simulink model "TEST_IPM_2_0"  (R2019b)
settings: configuration reference "Configuration" (kept outside this file)
PreLoadFcn:
  | RTWConfigurationCB('preloadfcn', bdroot);
values from neighbouring files (symbols this model uses):
  MParamFbase = 200.0    [TEST_IPM_LIB.sldd]
  MParamIbase = 360.0    [TEST_IPM_LIB.sldd]
  MParamLd = 8.0E-5    [TEST_IPM_LIB.sldd]
  MParamLq = 0.00028    [TEST_IPM_LIB.sldd]
  MParamRs = 0.014    [TEST_IPM_LIB.sldd]
  PWM_TPBRD_HALF = 5000.0    [TEST_IPM_LIB.sldd]
  Ts_10kHz = 0.0001    [TEST_IPM_LIB.sldd]
  Ts_1kHz = 0.001    [TEST_IPM_LIB.sldd]
undefined symbols (not defined in the file or in its folder): DiscIntNeverNeededParam, Down, GPTRIP1SEL, GPTRIP2SEL, TZ1, TZ2, Up
libraries: c280xlib x24, c2837xDlib x18, dsparch4 x11, c2802xlib x10, powerlib_meascontrol x9, dspstat3 x2, c2000lib x1, c2806xlib x1, idelinklib_common x1
(part 6 of 6)

== matlab function TEST_IPM_2_0/INT/Data Buffer/MATLAB Function ==
  data: IdREF input; IdFBK input; UdComP input; IqREF input; IqFBK input; UqComP input; Theta input; ArrayId_REF data_store_memory; ArrayId_FBK data_store_memory; ArrayIq_REF data_store_memory; ArrayIq_FBK data_store_memory; ArrayUdComP data_store_memory; ArrayUqComP data_store_memory; ArrayTheta data_store_memory; BufferFlag data_store_memory
function Buffer_In(IdREF,IdFBK,UdComP,IqREF,IqFBK,UqComP,Theta)
global ArrayId_REF ArrayId_FBK ArrayUdComP 
global ArrayIq_REF ArrayIq_FBK ArrayUqComP
global ArrayTheta
global BufferFlag
persistent count
if isempty(count)
	count = uint16(1);
end

if(BufferFlag == 1)
    count = uint16(1);
else
    if(count <= uint16(500))
        ArrayId_REF(count) = single(IdREF);
        ArrayId_FBK(count) = single(IdFBK);
        ArrayUdComP(count) = single(UdComP);
        ArrayIq_REF(count) = single(IqREF);
        ArrayIq_FBK(count) = single(IqFBK);
        ArrayUqComP(count) = single(UqComP);
        ArrayTheta (count) = single(Theta);
        count = count + uint16(1);
    else
        count = uint16(1);
        BufferFlag = uint16(1);
    end
end
end

== stateflow chart TEST_IPM_2_0/INT/MAX5742/MAX5742 ==
  settings: updateMethod=DISCRETE  initializeOutput=1  enableNonTerminalStates=1
  state DAC_A
    entry:
    count_5742 = uint16(0);
    DAC_A_OUT();
  state Wait
    entry:
    count_5742 = count_5742 + uint16(1);
  state DAC_B
    entry:
    count_5742 = uint16(0);
    DAC_B_OUT();
  state empty
  state Wait1
    entry:
    count_5742 = count_5742 + uint16(1);
  state DAC_C
    entry:
    count_5742 = uint16(0);
    DAC_C_OUT();
  state Wait3
    entry:
    count_5742 = count_5742 + uint16(1);
  state DAC_D
    entry:
    FLAG_5742 = uint16(1);
    count_5742 = uint16(0);
    DAC_D_OUT();
  (default) -> DAC_A
  empty -> DAC_A : [FLAG_5742 == 0]
  DAC_A -> (junction 5)
  (junction 5) -> Wait [order 2]
  Wait -> (junction 5)
  (junction 5) -> DAC_B [order 1] : [count_5742 > 20]
  DAC_B -> (junction 15)
  DAC_D -> empty
  (junction 15) -> Wait1 [order 2]
  Wait1 -> (junction 15)
  (junction 15) -> DAC_C [order 1] : [count_5742 > 20]
  DAC_C -> (junction 34)
  (junction 34) -> Wait3 [order 2]
  Wait3 -> (junction 34)
  (junction 34) -> DAC_D [order 1] : [count_5742 > 20]
  data: count_5742 data_store_memory; FLAG_5742 data_store_memory
  events: DAC_A_OUT output FUNCTION_CALL_EVENT; DAC_B_OUT output FUNCTION_CALL_EVENT; DAC_C_OUT output FUNCTION_CALL_EVENT; DAC_D_OUT output FUNCTION_CALL_EVENT

== matlab function TEST_IPM_2_0/INT/MAX5742/MAX1 ==
  events: DACA output FUNCTION_CALL_EVENT; DACB output FUNCTION_CALL_EVENT; DACC output FUNCTION_CALL_EVENT; DACD output FUNCTION_CALL_EVENT
function MAX5742
persistent count
if isempty(count)
	count = uint16(1);
end
count = count + uint16(1);
if(count == 1)
    DACA;
elseif(count == 2)
    DACB;
elseif(count == 3)
    DACC;
else
    count = uint16(0);
    DACD;
end
end

== matlab function TEST_IPM_2_0/INT/Extra Observer/MATLAB Function2 ==
  data: Z1 input; X1_hat output; X2_hat output; Z2 input; u1 input; u2 input; Theta1_hat output; Theta2_hat output; Theta3_hat output; Theta4_hat output; we input; weh input; Phid0 input; Phiq0 input; DEKF_R input; DEKF_Qx input; DEKF_QpRs input; DEKF_QpLdd input; DEKF_QpLdq input; DEKF_QpLqq input; DEKF_Clear input; INITV_RS data_store_memory; INITV_NDQ data_store_memory; INITV_NDD data_store_memory; INITV_NQQ data_store_memory
function [X1_hat,X2_hat,Theta1_hat,Theta2_hat,Theta3_hat,Theta4_hat] = EKF_ParameterObserver(Z1,Z2,u1,u2,we,weh,Phid0,Phiq0,DEKF_R,DEKF_Qx,DEKF_QpRs,DEKF_QpLdd,DEKF_QpLdq,DEKF_QpLqq,DEKF_Clear)
global INITV_RS INITV_NDD INITV_NDQ INITV_NQQ

persistent X_hat Theta_hat P_Theta_hat P_X_hat;
if isempty(X_hat)
    X_hat = single([0;0]);
end
if isempty(Theta_hat)
    Theta_hat = single([INITV_RS;INITV_NDD;INITV_NDQ;INITV_NQQ]) ;
end
if isempty(P_Theta_hat)
    P_Theta_hat = single(zeros(4));
end
if isempty(P_X_hat)
    P_X_hat = single(zeros(2));
end

persistent difX_difTheta K_xk_1 difH_difTheta;
if isempty(difX_difTheta)
    difX_difTheta =single(zeros(2,4));
end
if isempty(K_xk_1)
    K_xk_1 = single(zeros(2,2));
end
if isempty(difH_difTheta)
    difH_difTheta = single(zeros(2,4));
end
if(DEKF_Clear == uint16(1))
    X_hat = single([0;0]);
    Theta_hat = single([INITV_RS;INITV_NDD;INITV_NDQ;INITV_NQQ]) ;
    P_Theta_hat = single(zeros(4));
    P_X_hat = single(zeros(2));
    difX_difTheta =single(zeros(2,4));
    K_xk_1 = single(zeros(2,2));
    difH_difTheta = single(zeros(2,4));
end
U = [u1;u2];
Z = [Z1;Z2];
Ts = single(1e-4);
Qx = single([DEKF_Qx,0;0,DEKF_Qx]);
Qp = single(diag([DEKF_QpRs DEKF_QpLdd DEKF_QpLdq DEKF_QpLqq]));
R  = [DEKF_R,0;0,DEKF_R];
J = single([0 -1;1 0]);
%Step1: Parameter Prioi Estimation
Theta_PE = Theta_hat;
P_Theta_PE = P_Theta_hat + Qp;
%Step2: State Prioi Estimation
Rs = Theta_PE(1,1) * single(eye(2));
T = [Theta_PE(4,1),Theta_PE(3,1);Theta_PE(3,1),Theta_PE(2,1)];
% Phi = (single(eye(2)) + Ts .* (we * J - Rs * T));

A = -(we * J + Rs * T);
Phi = single(eye(2)) + A * Ts + single(0.5) * A^2 * Ts^2;
% Phi = eye(2) + Ts_EKF*A;
G = Ts *( single(eye(2)) + single(0.5) * A * Ts);
% G = Ts_EKF *( eye(2));

X_PE = Phi * X_hat + G * U - weh * J * Ts * [Phid0;Phiq0;];
P_X_PE = Phi * P_X_hat * Phi' + Qx;
%Step3: State Kalman Gain
K_xk = P_X_PE * T' * (T * P_X_PE * T' + R)^-1;
P_X_hat = (single(eye(2)) - K_xk * T) * P_X_PE;
%Step4: Parameter Kalman Gain
difX_hat_difTheta = difX_difTheta - K_xk_1 * difH_difTheta;
difF_difTheta = -Ts .* [Theta_hat(4,1) * X_hat(1) + Theta_hat(3,1) * X_hat(2),0,                        Theta_hat(1,1) * X_hat(2),Theta_hat(1,1) * X_hat(1);...
                        Theta_hat(3,1) * X_hat(1) + Theta_hat(2,1) * X_hat(2),Theta_hat(1,1) * X_hat(2),Theta_hat(1,1) * X_hat(1),0                        ;];
difF_difTheta = difF_difTheta + Phi * difX_hat_difTheta;
H_pk = [0,0,X_PE(2),X_PE(1);0,X_PE(2),X_PE(1),0] + T * difF_difTheta;

K_pk = P_Theta_PE * H_pk' * (H_pk * P_Theta_PE * H_pk' + R)^-1;
P_Theta_hat = (single(eye(4)) - K_pk * H_pk) * P_Theta_PE;
%Step5: State & Parameter Prediction
X_hat = X_PE + K_xk * (Z - T * X_PE);
Theta_hat = Theta_PE + K_pk * (Z - T * X_PE);
if(Theta_hat(1,1) > 0.01*100)
    Theta_hat(1,1) = single(0.01*100);
elseif (Theta_hat(1,1) < 0.01/100)
    Theta_hat(1,1) = single(0.01/100);
end
if(Theta_hat(2,1) > 3.8574*1e3*100)
    Theta_hat(2,1) = single(3.8574*1e3*100);
elseif (Theta_hat(2,1) < 3.8574*1e3/100)
    Theta_hat(2,1) = single(3.8574*1e3/100);
end
if(Theta_hat(3,1) > 448 * 100)
    Theta_hat(3,1) =  single(448 * 100);
elseif (Theta_hat(3,1) <  -448 * 100)
    Theta_hat(3,1) =  single(-448 * 100);
end
if(Theta_hat(4,1) > 1.2556*1e4*100)
    Theta_hat(4,1) = single(1.2556*1e4*100);
elseif (Theta_hat(4,1) < 1.2556*1e4/100)
    Theta_hat(4,1) = single(1.2556*1e4/100);
end
%Step6: Update the Parameter Kalman Gain
difX_difTheta = difF_difTheta;
K_xk_1 = K_xk;
difH_difTheta = H_pk;
if(DEKF_Clear == uint16(1))
    X_hat = single([0;0]);
    Theta_hat = single([INITV_RS;INITV_NDD;INITV_NDQ;INITV_NQQ]) ;
    P_Theta_hat = single(zeros(4));
    P_X_hat = single(zeros(2));
    difX_difTheta =single(zeros(2,4));
    K_xk_1 = single(zeros(2,2));
    difH_difTheta = single(zeros(2,4));
end
X1_hat = X_hat(1,1);X2_hat = X_hat(2,1);
Theta1_hat = Theta_hat(1,1);Theta2_hat = Theta_hat(2,1);Theta3_hat = Theta_hat(3,1);Theta4_hat = Theta_hat(4,1);

end

== matlab function TEST_IPM_2_0/INT/Extra Observer/MATLAB Function10 ==
  data: A input; Ldd output; B input; C input; Ldq output; Lqq output
function [Ldd,Ldq,Lqq] = inverse(A,B,C)
T = [C,B;B,A];
V = T^-1;
Ldd = V(1,1);
Ldq = V(1,2);
Lqq = V(2,2);
end

== matlab function TEST_IPM_2_0/INT/Extra Observer/MATLAB Function ==
  data: x1_hat input; idh output; x2_hat input; Ldd input; Ldq input; Lqq input; iqh output
function [idh,iqh] = OutputMatrix(x1_hat,x2_hat,Ldd,Ldq,Lqq)
X = [x1_hat;x2_hat];
L = [Ldd,Ldq;Ldq,Lqq];
Y = L * X;
idh = Y(1,1);
iqh = Y(2,1);
end

== matlab function TEST_IPM_2_0/INT/Motor Control/FbLMode/MATLAB Function1 ==
  data: udc_dem input; y output; Rdc input; speed input; Rs_norm input; Phi_dm_norm input; Lq_norm input; Cdc_norm input; iq_muti input
function y = fcn(udc_dem,Rdc, speed, Rs_norm, Phi_dm_norm, Lq_norm, Cdc_norm,iq_muti)
we = speed*2*pi/60*4;
a = Rs_norm;
b = we*Phi_dm_norm;
c = 2/3*udc_dem*udc_dem/Rdc;
iq = (-b+sqrt(abs(b*b-4*a*c)))/2/a;
y = 3*Lq_norm*iq*iq/2*iq_muti+Cdc_norm*udc_dem*udc_dem;

== matlab function TEST_IPM_2_0/Temperature&DCBUS/MATLAB Function5 ==
  events: fcncall output FUNCTION_CALL_EVENT
function fcn
fcncall

== matlab function TEST_IPM_2_0/INT/Motor Control/TorqueMode/Current_PI1/MATLAB Function5 ==
  data: Imd input; idh output; Imq input; FRQ input; iqh output
function [idh,iqh] = HFI(Imd,Imq,FRQ)
persistent HFI_COUNT
if isempty(HFI_COUNT)
    HFI_COUNT = single(0);
end
HFI_COUNT = HFI_COUNT + single(2)*single(pi)*single(1e-4)*FRQ;
if(HFI_COUNT >= single(2)*single(pi))
    HFI_COUNT = HFI_COUNT - single(2)*single(pi);
end

idh = Imd * sin (HFI_COUNT);
iqh = Imq * cos (HFI_COUNT);

== matlab function TEST_IPM_2_0/Temperature&DCBUS/Function-Call Subsystem1/MATLAB Function5 ==
  data: Id_Sam input; Tr_Calk1 output; Iq_Sam input; Speed_Sam input; Ts input; Tr_Calk0 input; Ts_Calk0 input; Tw_Calk0 input; Tew_Calk0 input; Tb_Calk0 input; Tf_Sam input; Flowrate input; Ts_Calk1 output; Tw_Calk1 output; Tew_Calk1 output; Tb_Calk1 output; Tem_Cal output; Ps_Cal output; Pr_Cal output; Pw_Cal output; Pew_Cal output; Pb_Cal output; Faid_Cal output; Faiq_Cal output
function [Tr_Calk1,Ts_Calk1,Tw_Calk1,Tew_Calk1,Tb_Calk1,Tem_Cal,Ps_Cal,Pr_Cal,Pw_Cal,Pew_Cal,Pb_Cal,Faid_Cal,Faiq_Cal] = TempCal7_Realtime(Id_Sam,Iq_Sam,Speed_Sam,Ts,Tr_Calk0,Ts_Calk0,Tw_Calk0,Tew_Calk0,Tb_Calk0,Tf_Sam,Flowrate)
% 温度、转矩、磁链、损耗预测  
% 温度、转矩预测较准确
% 磁链、损耗计算值仅供参考

%   输入：
%       d轴采样电流 
%       q轴采样电流 
%       采样转速（rpm） 
%       采样周期 
%       Tr（转子）上一步计算值(0时刻初值赋冷却水温度) 
%       Ts（定子）上一步计算值 (0时刻初值赋冷却水温度)
%       Tw（槽内绕组）上一步计算值(0时刻初值赋冷却水温度)
%       Tew（端部绕组）上一步计算值(0时刻初值赋冷却水温度)
%       Tb（轴承）上一步计算值(0时刻初值赋冷却水温度) 
%       冷却水采样温度（Tf） 
%       冷却水流量
%   输出：
%       Tr（转子）当前计算值 
%       Ts（定子）当前计算值 
%       Tw（槽内绕组）当前计算值 
%       Tew（端部绕组）当前计算值  
%       Tb（轴承）当前计算值 
%       转矩
%       定子铁耗
%       转子损耗
%       槽内绕组损耗
%       端部绕组损耗
%       轴承摩擦损耗
%       d轴磁链
%       q轴磁链


%% 电机相关参数
Kdp1=0.9298;    %基波绕组系数
afi=0.636619772367581;
N_ph=16;    %每相串联匝数
St1=7.83e-4;
St2=10e-4;      %齿部截面积
Sy=0.002;
Vt1=9.2832e-4;  
Vt2=8.896128e-05;   %齿部体积
Vy=0.0013587424;
Soft_rou=7600;  %铁心密度
Z=48;
p=4;    %极对数

%% 辨识参数值
Para_id=[0.0580952329317469;-0.00118000000000000;0.0599996256179708;0.00102365041716703;-0.0100098006875944;-0.00199999089944106;-0.0199976933846070;0.176564851799861;-0.116369689538171;-0.00699999983189507;7.92416366396190e-05;-1.36108306558421e-06;-3.99997706572135e-05;3.99998410778491e-05;0.0261290991243893;-1.11391676740694e-05;0.0765120005266704;0.413720950349751;1.57193023256519e-05;3.68281568448212e-05;0.982247624109508;0.00439999995944245;0.00386261247030165;0.838544964265891;0.639998220239094;2;1.99997523947852;1.06112673905865;21.9998787199779;0.300235749665813;0.800000000104399;0.300002824107786;3.99994869235477;0.126723044416704;0.0189694146075085;0.799998239086721;0.0204336063545049;0.0130758077128373;0.799999907234451;0.0645185779172808;0.799998992255128;2547.20014686192;3252.41687571480;847.622925348872;3376.43780564643;973.528304341396;0.500000357788724;0.500248365159868;0.200610877247107;3.99998864460978;4.99996291200200];
%d磁链
Fai_PM0=Para_id(1);         %T0温度 空载永磁磁链幅值 FEA@60C,0.061304 0.05946  (0.05941, 0.05951)
Fai_PMafi=Para_id(2);       %剩磁温度系数,-0.0012
Fd_k1=Para_id(3);           %多项式系数0.0532  (0.05298, 0.05342)
Fd_k2=Para_id(4);           %0.002669  (0.002441, 0.002896)
Fd_k3=Para_id(5);           %-0.01527  (-0.01553, -0.01501)
Fd_k4=Para_id(6);           %-0.001465  (-0.001751, -0.001178)
Fd_k5=Para_id(7);           %-0.01125  (-0.01155, -0.01096)
%q磁链
Fq_k1=Para_id(8);           %多项式系数0.1824  (0.182, 0.1828)
Fq_k2=Para_id(9);           %-0.1385  (-0.1396, -0.1374)
Fq_k3=Para_id(10);          %-0.005672  (-0.006335, -0.005008)
%铁耗
ke_k1=Para_id(11);          %ke多项式系数7.356e-05  (7.204e-05, 7.507e-05)
ke_k2=Para_id(12);          %-0.0001235  (-0.0001265, -0.0001205)
ke_k3=Para_id(13);          %-1.666e-05  (-1.803e-05, -1.529e-05)
ke_k4=Para_id(14);          %1.683e-05  (1.441e-05, 1.924e-05)
kh_k1=Para_id(15);          %kh多项式系数0.02411  (0.02377, 0.02445)
kh_k2=Para_id(16);          %-0.0134  (-0.014, -0.01281)
kh_k3=Para_id(17);          %0.1388  (0.1374, 0.1401)
ks1=Para_id(18);            %定子铁耗占总铁耗比例的系数ks,0.4-0.8
ks2=Para_id(19);            %0-0.2
ks3=Para_id(20);            %0-0.2
ks4=Para_id(21);            %0-0.2
%铜耗
Rs0=Para_id(22);            %T0温度相电阻,21.5度,0.004213333 
Rsafi=Para_id(23);          %铜温度系数,0.003862-0.00404
Rsbeta=Para_id(24);         %Rac/Rdc随温度变化系数,0.83,0.5-1,0-3
kw0=Para_id(25);            %槽内绕组占比,0.633802 ,0.6-0.65
kw1=Para_id(26);            %Rac/Rdc系数,0-2,
kw2=Para_id(27);            %Rac/Rdc系数,0-2,
%轴承损耗
kb=Para_id(28);             %1-3
%端部对流热阻
k1_hew=Para_id(29);         %14-24
k2_hew=Para_id(30);         %0.35-0.5
k3_hew=Para_id(31);         %0.9-1
EwAir_pu=Para_id(32);   %端部空气流速标幺值,相对于转子表面速0.4-0.8
Rew_endair_co=Para_id(33);        
%常值热阻
Rrs_C=Para_id(34);          % 0.019037   0.056793 
Rsf_C=Para_id(35);          %0.011580 	0.058256
Rrb_C=Para_id(36);          %0.147759 	0.221187 
Rsw_C=Para_id(37);          %0.010558 	0.036469
Rwew_C=Para_id(38);         %0.037152 	0.054677
Rewf_C=Para_id(39);         %0.194390   0.310690
Rbf_C=Para_id(40);          %1.200250 	2.358350 ]
Rrf_C=Para_id(41);
%常值热容
Cr_C=Para_id(42);
Cs_C=Para_id(43);
Cw_C=Para_id(44);
Cew_C=Para_id(45);
Cb_C=Para_id(46);
%修正系数
Rrs_co=Para_id(47);
%
RAir_pu=Para_id(48);             %转子端部空气流速标幺值
CapHouseAir_pu=Para_id(49);    %端盖机壳内表面空气流速标幺值
Rr_endair_co=Para_id(50);
Rendair_housecap_co=Para_id(51);

%% 标幺值
Fd1_Sam=Speed_Sam*p/60;
Fd1_SamBy=Fd1_Sam/1000; %标幺     
Id_SamBy=Id_Sam/556;    %标幺值
Iq_SamBy=Iq_Sam/556;
Iamp_Sam=sqrt(Id_Sam.^2+Iq_Sam.^2);
Iamp_SamBy=Iamp_Sam/556;

%% 开始计算
%水套对流热阻
Water_v=7.904e-7;       %运动粘度m2/s，30°物性
Water_Pr=5.31;          %普朗特数
Water_Lamda=0.620;      %热导率
Water_Flow=Flowrate;          %流量L/min
Wj_C=0.07284955592;         %水道周长
Wj_SeS=0.00013627433;       %水道截面积
Wj_D=4*Wj_SeS/Wj_C;         %水力直径
Wj_S_act=0.13768566069;         %有效部分的水道接触面积
Wj_S_end=0.10912863477;         %机壳连接水道接触面积
Wj_Speed=Water_Flow/1000/60/Wj_SeS;
Wj_Re=Wj_Speed*Wj_D/Water_v;
Wj_f=(0.79*log(Wj_Re)-1.64)^-2;
Wj_Nu=Wj_f/8*(Wj_Re-1000)*Water_Pr/(1+12.7*(Wj_f/8)^0.5*(Water_Pr^(2/3)-1));
Wj_h=Wj_Nu*Water_Lamda/Wj_D;
R_Wj_act=1/(Wj_h*Wj_S_act);
R_Wj_end=1/(Wj_h*Wj_S_end);

%端部对流、气隙对流所需参数
Rsi=0.0725;
Rro=0.0717;
Airgap_g=Rsi-Rro;
Rotor_omega=2*pi*Speed_Sam/60;
Rotor_v=Rotor_omega*Rro;
%端部绕组-端部空气对流热阻
h_ew=k1_hew*(1+k2_hew*(EwAir_pu*Rotor_v)^k3_hew);
Rew_endair=Rew_endair_co*1/(h_ew*10.5e-2);        %EWS是两端绕组的对流面积
%转子端部_端部机壳对流热阻
hr_ew=k1_hew*(1+k2_hew*(RAir_pu*Rotor_v)^k3_hew);
Rr_endair=Rr_endair_co*1/(hr_ew*4.3784e-2);        %EWS是两端绕组的对流面积
%端部空气-端盖机壳对流热阻
hew_caphouse=k1_hew*(1+k2_hew*(CapHouseAir_pu*Rotor_v)^k3_hew);
Rair_caphouse=Rendair_housecap_co*1/(hew_caphouse*15.08e-2);        %EWS是两端绕组的对流面积

%气隙对流热阻
Air_gap_rm=0.5*(Rro+Rsi);
Air_gap_rlog=(Rsi-Rro)/log(Rsi/Rro);
Air_gap_v=18.9e-6;      %运动粘度m2/s
Air_gap_k=0.02803;
Air_gap_S=0.0571*(1-0.652*(Rsi-Rro)/Rro)+0.00056*(1-0.652*(Rsi-Rro)/Rro)^(-1);
Air_gap_Fg=pi^2/sqrt(Air_gap_S)/41.19*(1-(Rsi-Rro)/(2*Air_gap_rm))^(-1);
Tam=Rotor_omega*Air_gap_rm^0.5*(Rsi-Rro)^1.5/Air_gap_v;
Tam2_Fg2=Tam^2/Air_gap_Fg^2;
if Tam2_Fg2 <1700
    Nu_Airgap =single(2*(Rsi-Rro)/Rro/log(1+(Rsi-Rro)/Rro));
elseif Tam2_Fg2 >=1700&&Tam2_Fg2 <1e4
    Nu_Airgap =single(0.128*Tam2_Fg2 ^0.367);
elseif Tam2_Fg2 >=1e4&&Tam2_Fg2 <1e7
    Nu_Airgap =single(0.409*Tam2_Fg2 ^0.241); 
else
    Nu_Airgap = single(0.409*Tam2_Fg2 ^0.241);
end
h_Airgap =Nu_Airgap *Air_gap_k/(2*Airgap_g);
R_Airgap =1/(h_Airgap *2*pi*Air_gap_rlog*0.135);    %定子内表面到转子外表面的对流热阻
%Rrs热阻更新
Rrs =(R_Airgap +Rrs_C)*Rrs_co;Grs =1/Rrs ;

%低阶热网络热阻热容
Rsf=(R_Wj_act+Rsf_C);Gsf=1/Rsf; %0.000510116309968285+(0.011580 	0.058256 )
Rrb=Rrb_C;Grb=1/Rrb;        %0.147759 	0.221187 
Rsw=Rsw_C;Gsw=1/Rsw;        %0.010558 	0.036469 
Rwew=Rwew_C;Gwew=1/Rwew;	%0.037152 	0.054677 
Rbf=Rbf_C;Gbf=1/Rbf;        %1.200250 	2.358350 
Rewf =Rew_endair +Rair_caphouse +R_Wj_end+Rewf_C;Gewf =1/Rewf ;
Rrf =Rr_endair +Rair_caphouse +R_Wj_end+Rrf_C;Grf =1/Rrf ;
Cr=Cr_C ;
Cs=Cs_C ;
Cw=Cw_C ;
Cew=Cew_C ;
Cb=Cb_C ;

%磁链计算
Fai_PM =Fai_PM0*(1+Fai_PMafi*(Tr_Calk0 -20));
Faid_Cal =Fai_PM +Fd_k1*Id_SamBy +Fd_k2*abs(Iq_SamBy )+Fd_k3*Id_SamBy *abs(Iq_SamBy )+Fd_k4*Id_SamBy ^2+Fd_k5*Iq_SamBy ^2;
Faiq_Cal =Fq_k1*Iq_SamBy +Fq_k2*Iq_SamBy ^3+Fq_k3*Id_SamBy *Iq_SamBy ;
Faiamp =sqrt(Faid_Cal ^2+Faiq_Cal ^2);
%定子磁密计算
Bmt1 =2*p*Faiamp /(afi*N_ph*Kdp1*St1*Z);         %齿部平均磁密
Bmt2 =2*p*Faiamp /(afi*N_ph*Kdp1*St2*Z);         %齿尖平均磁密
Bmy =Faiamp /(2*N_ph*Kdp1*Sy);
%定子铁耗计算
ket1 =ke_k1+ke_k2*Bmt1 /2+ke_k3*Fd1_SamBy +ke_k4*Bmt1 /2*Fd1_SamBy ;
kht1 =kh_k1+kh_k2*Bmt1 /2+kh_k3*Fd1_SamBy *(Bmt1 /2)^2;
pfest1 =(ket1 *Fd1_SamBy +kht1 )*Fd1_Sam *Bmt1 ^2;
Pfest1 =pfest1 *Vt1*Soft_rou;   %齿部铁耗     
ket2 =ke_k1+ke_k2*Bmt2 /2+ke_k3*Fd1_SamBy +ke_k4*Bmt2 /2*Fd1_SamBy ;
kht2 =kh_k1+kh_k2*Bmt2 /2+kh_k3*Fd1_SamBy *(Bmt2 /2)^2;
pfest2 =(ket2 *Fd1_SamBy +kht2 )*Fd1_Sam *Bmt2 ^2;
Pfest2 =pfest2 *Vt2*Soft_rou;   %齿尖铁耗 
key =ke_k1+ke_k2*Bmy /2+ke_k3*Fd1_SamBy +ke_k4*Bmy /2*Fd1_SamBy ;
khy =kh_k1+kh_k2*Bmy /2+kh_k3*Fd1_SamBy *(Bmy /2)^2;
pfesy =(key *Fd1_SamBy +khy )*Fd1_Sam *Bmy ^2;
Pfesy =pfesy *Vy*Soft_rou;
Pfes =Pfest1 +Pfest2 +Pfesy ;
Ps_Cal =Pfes ;
%转子铁耗计算（含磁钢损耗）
ks =ks1+ks2*Iamp_SamBy +ks3*Fd1_SamBy +ks4*Iamp_SamBy *Fd1_SamBy ;
Pfer =(1-ks )*Pfes/ks;
Pr_Cal =Pfer ;
%槽内铜耗计算
Rcu_wT0 =kw0*Rs0;                                 %槽内直流电阻（T0温度）
Rcu_ewT0 =(1-kw0)*Rs0;                            %端部直流电阻（T0温度）
Rcu_wT =Rcu_wT0 *(1+Rsafi*(Tw_Calk0 -15));      %槽内直流电阻温度修正
Rcu_ewT =Rcu_ewT0 *(1+Rsafi*(Tew_Calk0 -15));   %端部直流电阻温度修正
Ratio_RwT0 =1+kw1*(Fd1_SamBy )+kw2*(Fd1_SamBy )^2;                    %槽内的Rac/Rdc（T0温度），端部不考虑交流效应
Ratio_RwT =1+(Ratio_RwT0 -1)/( 1+Rsafi*(Tw_Calk0 -15)^(Rsbeta+1) );     %槽内的Rac/Rdc温度修正，端部不考虑交流效应
Pw_Cal =3/2*Iamp_Sam ^2*Rcu_wT *Ratio_RwT ;       %槽内绕组铜耗
Pew_Cal =3/2*Iamp_Sam ^2*Rcu_ewT ;                  %端部绕组铜耗
%轴承损耗
Pb_Cal =kb*0.03*(20)*Rotor_omega /pi;

%计算温度
Mat_Cap=diag([Cr ,Cs ,Cw ,Cew ,Cb ]);     %热容矩阵
Mat_Con=[Grs+Grb+Grf ,            -Grs,              0,                  0,              -Grb 
        -Grs ,              Grs+Gsw+Gsf ,             -Gsw ,            0,                    0
        0,                          -Gsw ,              Gsw+Gwew ,     -Gwew ,                0
        0,                          0,                  -Gwew ,           Gwew+Gewf ,          0
        -Grb ,                    0,                      0,                  0,           Grb+Gbf ];     %热导矩阵
Mat_Bsubsub=[   0,      Grf 
                0,      Gsf 
                0,      0
                0,      Gewf 
                0,      Gbf ];
Mat_Bsub=[eye(5),Mat_Bsubsub];
Mat_A=Mat_Cap^(-1)*(-Mat_Con);         %状态矩阵
Mat_B=Mat_Cap^(-1)*Mat_Bsub;        %输入矩阵
Mat_u=[Pr_Cal ,Ps_Cal ,Pw_Cal ,Pew_Cal ,Pb_Cal ,20 ,Tf_Sam ]';   %控制向量
Tmat_Calk0=[Tr_Calk0,Ts_Calk0,Tw_Calk0,Tew_Calk0,Tb_Calk0]';
Tmat_Calk1=Ts*( Mat_A*Tmat_Calk0+Mat_B*Mat_u )+Tmat_Calk0;   
Tr_Calk1=Tmat_Calk1(1);
Ts_Calk1=Tmat_Calk1(2);
Tw_Calk1=Tmat_Calk1(3);
Tew_Calk1=Tmat_Calk1(4);
Tb_Calk1=Tmat_Calk1(5);

%转矩计算
Tem_Cal=3/2*p*(Faid_Cal*Iq_Sam-Faiq_Cal*Id_Sam);

end

== matlab function TEST_IPM_2_0/INT/GPIO UP/MATLAB Function2 ==
  data: IGBT_FAULT input; STOP data_store_memory; PROTECT data_store_memory
function DRIVE_FAULT(IGBT_FAULT)
global STOP PROTECT
if (IGBT_FAULT ~= uint16(63))
    STOP = uint16(1);
     PROTECT = uint16(bitor(PROTECT,uint16(32)));
end

== matlab function TEST_IPM_2_0/INT/Motor Control/Current_PI/MATLAB Function4 ==
  data: Frq input
  events: FilterEnable output FUNCTION_CALL_EVENT
function FILTER_ENABLE(Frq)
    if(Frq > 0)
        FilterEnable();
    end
end

== matlab function TEST_IPM_2_0/INT/Motor Control/TorqueMode/MATLAB Function2 ==
  data: Target input; Set_Point output; Step input; STOP data_store_memory
function Set_Point = RAMP_Control(Target,Step)
global STOP;

persistent Set_Point_Value;
if isempty(Set_Point_Value)
   Set_Point_Value = single(0);
end
if(Target >= Set_Point_Value)
	Set_Point_Value = Set_Point_Value + Step;
else
	Set_Point_Value = Set_Point_Value - Step;
end


if(abs(Target - Set_Point_Value) <= Step*2)
    Set_Point_Value = Target;
end


if(Set_Point_Value >= single(400))
    Set_Point_Value = single(400);
elseif(Set_Point_Value <= single(-400))
    Set_Point_Value = single(-400);
end
if(STOP ~= uint16(0))
    Set_Point_Value = single(0);
end
Set_Point = Set_Point_Value;
end

== matlab function TEST_IPM_2_0/INT/Read Rotor Position/SpeedCal/MATLAB Function1 ==
  data: theta input; speed output single; theta_old input; Ts_1kHz parameter
function speed = Est_Speed(theta,theta_old, Ts_1kHz)

error = (theta - theta_old);
if(error > pi)
    error = error - single(2)*single(pi);
elseif(error <- pi)
	error = error + single(2)*single(pi);
end
speed = error/(Ts_1kHz)*single(9.54929674)*single(0.25);
end

== matlab function TEST_IPM_2_0/INT/Motor Control/TorqueMode/MATLAB Function1 ==
  data: n input
  events: PI_Clear output FUNCTION_CALL_EVENT
function n_Protect(n)

    if(n < -50)
        PI_Clear;
    end
end

== matlab function TEST_IPM_2_0/INT/Motor Control/TorqueMode/Current_PI1/MATLAB Function6 ==
  data: IRef input; IFbk input; PROTECT data_store_memory; STOP data_store_memory
function DQCurrentProtect(IRef,IFbk)
global PROTECT STOP
if(abs(IRef - IFbk) >= 150)
    STOP = uint16(1);
    PROTECT = uint16(bitor(PROTECT,16)); 
end    
if(PROTECT ~= uint16(0))
    STOP = uint16(1);
end

== matlab function TEST_IPM_2_0/INT/Motor Control/TorqueMode/Current_PI1/MATLAB Function7 ==
  data: IRef input; IFbk input; PROTECT data_store_memory; STOP data_store_memory
function DQCurrentProtect(IRef,IFbk)
global PROTECT STOP
if(abs(IRef - IFbk) >= 150)
    STOP = uint16(1);
    PROTECT = uint16(bitor(PROTECT,16)); 
end    
if(PROTECT ~= uint16(0))
    STOP = uint16(1);
end

== matlab function TEST_IPM_2_0/INT/Motor Control/Current_PI/DEKF_Filter/MATLAB Function1 ==
  data: theta input; speed output single; theta_old input
function speed = Est_Speed(theta,theta_old)

error = (theta - theta_old);
if(error > pi)
    error = error - single(2)*single(pi);
elseif(error <- pi)
	error = error + single(2)*single(pi);
end
speed = error*single(10e3)*single(9.54929674)*single(0.25);
end

== matlab function TEST_IPM_2_0/INT/Extra Observer/MATLAB Function1 ==
  data: idh input; X1_hat output; iqh input; udh input; uqh input; we0 input; weh input; Phid0 input; Phiq0 input; R input; Qx input; QpRs input; QpLdd input; QpLdq input; QpLqq input; X2_hat output; Theta1_hat output; Theta2_hat output; Theta3_hat output; Theta4_hat output; clear input; INITV_RS data_store_memory; INITV_NDQ data_store_memory; INITV_NDD data_store_memory; INITV_NQQ data_store_memory
function [X1_hat,X2_hat,Theta1_hat,Theta2_hat,Theta3_hat,Theta4_hat] = EKF(idh,iqh,udh,uqh,we0,weh,Phid0,Phiq0,R, Qx, QpRs,QpLdd,QpLdq,QpLqq,clear)
global INITV_RS INITV_NDD INITV_NDQ INITV_NQQ
persistent Pk1_k1 Xk1_k1;
if isempty(Pk1_k1)
    Pk1_k1 = single(zeros(6,6));
end
if isempty(Xk1_k1)
    Xk1_k1 = [single(0),single(0),INITV_RS,INITV_NDD,INITV_NDQ,INITV_NQQ]';
end

if(clear ==1)
    Xk1_k1 = [single(0),single(0),INITV_RS,INITV_NDD,INITV_NDQ,INITV_NQQ]';
    Pk1_k1 = single(zeros(6,6));
end
U = [udh;uqh];
Ih= [idh;iqh];
Pk0_k0 = Pk1_k1;
J = single([0,-1;1,0]);
I = single([1,0;0,1]);
Ts = single(1e-4);
Q = single(diag([Qx Qx QpRs QpLdd QpLdq QpLqq]));
R  = [R,0;0,R];
Rs = Xk1_k1(3,1) * I;
T = [Xk1_k1(6,1),Xk1_k1(5,1);...
     Xk1_k1(5,1),Xk1_k1(4,1);];
A = -(we0 * J + Rs * T);
Phi = I + A * Ts + single(0.5) * A^2 * Ts^2;
G = Ts * (I + single(0.5) * A * Ts);
X_hat = [Xk1_k1(1,1);Xk1_k1(2,1)];
X_PE = Phi * X_hat + G * U;
xk1_k0 = [X_PE(1,1);X_PE(2,1);Xk1_k1(3,1);Xk1_k1(4,1);Xk1_k1(5,1);Xk1_k1(6,1);];
Fk0 = [1 + Ts * xk1_k0(3,1) * xk1_k0(6,1),       Ts * (we0 + xk1_k0(3,1) * xk1_k0(5,1)),  Ts * xk1_k0(6,1) * Xk1_k1(1,1) + Ts * xk1_k0(5,1) * Xk1_k1(2,1), 0                             , Ts * xk1_k0(3,1) * Xk1_k1(2,1), Ts * xk1_k0(3,1) * Xk1_k1(1,1);...
       Ts * (-we0 + xk1_k0(3,1) * xk1_k0(5,1)),  1 + Ts * xk1_k0(3,1) * xk1_k0(4,1),      Ts * xk1_k0(5,1) * Xk1_k1(1,1) + Ts * xk1_k0(4,1) * Xk1_k1(2,1), Ts * xk1_k0(3,1) * Xk1_k1(2,1), Ts * xk1_k0(3,1) * Xk1_k1(1,1), 0                             ;...
       0,                                       0,                                      1,                                                               0,                              0,                                0                             ;...
       0,                                       0,                                      0,                                                               1,                              0,                                0                             ;...
       0,                                       0,                                      0,                                                               0,                              1,                                0                             ;...
       0,                                       0,                                      0,                                                               0,                              0,                                1                             ;];
E = Fk0(1:2,1:6) * Pk0_k0;
Temp = [E(1,1)      E(1,2)      E(1,3)      E(1,4)      E(1,5)      E(1,6)      ;...
        E(2,1)      E(2,2)      E(2,3)      E(2,4)      E(2,5)      E(2,6)      ;...
        Pk0_k0(3,1) Pk0_k0(3,2) Pk0_k0(3,3) Pk0_k0(3,4) Pk0_k0(3,5) Pk0_k0(3,6) ;...
        Pk0_k0(4,1) Pk0_k0(4,2) Pk0_k0(4,3) Pk0_k0(4,4) Pk0_k0(4,5) Pk0_k0(4,6) ;...
        Pk0_k0(5,1) Pk0_k0(5,2) Pk0_k0(5,3) Pk0_k0(5,4) Pk0_k0(5,5) Pk0_k0(5,6) ;...
        Pk0_k0(6,1) Pk0_k0(6,2) Pk0_k0(6,3) Pk0_k0(6,4) Pk0_k0(6,5) Pk0_k0(6,6) ;];
Pk1_k0 = Temp * Fk0 + Q;
yk1 = T * X_PE;
yk1Error = Ih - yk1;
Hk = [xk1_k0(6,1),xk1_k0(5,1),0,0,          xk1_k0(2,1),xk1_k0(1,1);...
      xk1_k0(5,1),xk1_k0(4,1),0,xk1_k0(2,1),xk1_k0(1,1),0          ;];
Sk = Hk * Pk1_k0 * Hk' + R;
Kk = Pk1_k0 * Hk' * (Sk^-1);
Xk1_k1 = xk1_k0 + Kk*yk1Error;
Pk1_k1 = (eye(6) - Kk * Hk) * Pk1_k0;

if(Xk1_k1(3,1) > 0.01*100)
    Xk1_k1(3,1) = single(0.01*100);
elseif (Xk1_k1(3,1) < 0.01/100)
    Xk1_k1(3,1) = single(0.01/100);
end
if(Xk1_k1(4,1) > 3.8574*1e3*100)
    Xk1_k1(4,1) = single(3.8574*1e3*100);
elseif (Xk1_k1(4,1) < 3.8574*1e3/100)
    Xk1_k1(4,1) = single(3.8574*1e3/100);
end
if(Xk1_k1(5,1) > 448 * 100)
    Xk1_k1(5,1) =  single(448 * 100);
elseif (Xk1_k1(5,1) <  -448 * 100)
    Xk1_k1(5,1) =  single(-448 * 100);
end
if(Xk1_k1(6,1) > 1.2556*1e4*100)
    Xk1_k1(6,1) = single(1.2556*1e4*100);
elseif (Xk1_k1(6,1) < 1.2556*1e4/100)
    Xk1_k1(6,1) = single(1.2556*1e4/100);
end
X1_hat = Xk1_k1(1,1);X2_hat = Xk1_k1(2,1);
Theta1_hat = Xk1_k1(3,1);Theta2_hat = Xk1_k1(4,1);Theta3_hat = Xk1_k1(5,1);Theta4_hat = Xk1_k1(6,1);

== matlab function TEST_IPM_2_0/INT/Extra Observer/MATLAB Function3 ==
  data: A input; Ldd output; B input; C input; Ldq output; Lqq output
function [Ldd,Ldq,Lqq] = inverse(A,B,C)
T = [C,B;B,A];
V = T^-1;
Ldd = V(1,1);
Ldq = V(1,2);
Lqq = V(2,2);
end

== matlab function TEST_IPM_2_0/INT/Extra Observer/MATLAB Function4 ==
  data: nRef input; Gamma output; Bias input
function Gamma = GammaComP(nRef,Bias)

Gamma = single(5.819e-6) * nRef + Bias;

== matlab function TEST_IPM_2_0/Subsystem1/MATLAB Function1 ==
  data: idh input; X1_hat output; iqh input; udh input; uqh input; we0 input; weh input; Phid0 input; Phiq0 input; R input; Qx input; QpRs input; QpLdd input; QpLdq input; QpLqq input; X2_hat output; Theta1_hat output; Theta2_hat output; Theta3_hat output; Theta4_hat output; clear input; INITV_RS data_store_memory; INITV_NDQ data_store_memory; INITV_NDD data_store_memory; INITV_NQQ data_store_memory
function [X1_hat,X2_hat,Theta1_hat,Theta2_hat,Theta3_hat,Theta4_hat] = EKF(idh,iqh,udh,uqh,we0,weh,Phid0,Phiq0,R, Qx, QpRs,QpLdd,QpLdq,QpLqq,clear)
global INITV_RS INITV_NDD INITV_NDQ INITV_NQQ
persistent Pk1_k1 Xk1_k1;
if isempty(Pk1_k1)
    Pk1_k1 = single(zeros(6,6));
end
if isempty(Xk1_k1)
    Xk1_k1 = [single(0),single(0),INITV_RS,INITV_NDD,INITV_NDQ,INITV_NQQ]';
end

if(clear ==1)
    Xk1_k1 = [single(0),single(0),INITV_RS,INITV_NDD,INITV_NDQ,INITV_NQQ]';
    Pk1_k1 = single(zeros(6,6));
end
U = [udh;uqh];
Ih= [idh;iqh];
Pk0_k0 = Pk1_k1;
J = single([0,-1;1,0]);
I = single([1,0;0,1]);
Ts = single(5e-4);
Q = single(diag([Qx Qx QpRs QpLdd QpLdq QpLqq]));
R  = [R,0;0,R];
Rs = Xk1_k1(3,1) * I;
T = [Xk1_k1(6,1),Xk1_k1(5,1);...
     Xk1_k1(5,1),Xk1_k1(4,1);];
A = -(we0 * J + Rs * T);
Phi = I + A * Ts + single(0.5) * A^2 * Ts^2;
G = Ts * (I + single(0.5) * A * Ts);
X_hat = [Xk1_k1(1,1);Xk1_k1(2,1)];
X_PE = Phi * X_hat + G * U;
xk1_k0 = [X_PE(1,1);X_PE(2,1);Xk1_k1(3,1);Xk1_k1(4,1);Xk1_k1(5,1);Xk1_k1(6,1);];
Fk0 = [1 + Ts * xk1_k0(3,1) * xk1_k0(6,1),       Ts * (we0 + xk1_k0(3,1) * xk1_k0(5,1)),  Ts * xk1_k0(6,1) * Xk1_k1(1,1) + Ts * xk1_k0(5,1) * Xk1_k1(2,1), 0                             , Ts * xk1_k0(3,1) * Xk1_k1(2,1), Ts * xk1_k0(3,1) * Xk1_k1(1,1);...
       Ts * (-we0 + xk1_k0(3,1) * xk1_k0(5,1)),  1 + Ts * xk1_k0(3,1) * xk1_k0(4,1),      Ts * xk1_k0(5,1) * Xk1_k1(1,1) + Ts * xk1_k0(4,1) * Xk1_k1(2,1), Ts * xk1_k0(3,1) * Xk1_k1(2,1), Ts * xk1_k0(3,1) * Xk1_k1(1,1), 0                             ;...
       0,                                       0,                                      1,                                                               0,                              0,                                0                             ;...
       0,                                       0,                                      0,                                                               1,                              0,                                0                             ;...
       0,                                       0,                                      0,                                                               0,                              1,                                0                             ;...
       0,                                       0,                                      0,                                                               0,                              0,                                1                             ;];
Pk1_k0 = Fk0 * Pk0_k0 * Fk0' + Q;
yk1 = T * X_PE;
yk1Error = Ih - yk1;
Hk = [xk1_k0(6,1),xk1_k0(5,1),0,0,          xk1_k0(2,1),xk1_k0(1,1);...
      xk1_k0(5,1),xk1_k0(4,1),0,xk1_k0(2,1),xk1_k0(1,1),0          ;];
Sk = Hk * Pk1_k0 * Hk' + R;
Kk = Pk1_k0 * Hk' * (Sk^-1);
Xk1_k1 = xk1_k0 + Kk*yk1Error;
Pk1_k1 = (eye(6) - Kk * Hk) * Pk1_k0;

if(Xk1_k1(3,1) > 0.01*100)
    Xk1_k1(3,1) = single(0.01*100);
elseif (Xk1_k1(3,1) < 0.01/100)
    Xk1_k1(3,1) = single(0.01/100);
end
if(Xk1_k1(4,1) > 3.8574*1e3*100)
    Xk1_k1(4,1) = single(3.8574*1e3*100);
elseif (Xk1_k1(4,1) < 3.8574*1e3/100)
    Xk1_k1(4,1) = single(3.8574*1e3/100);
end
if(Xk1_k1(5,1) > 448 * 100)
    Xk1_k1(5,1) =  single(448 * 100);
elseif (Xk1_k1(5,1) <  -448 * 100)
    Xk1_k1(5,1) =  single(-448 * 100);
end
if(Xk1_k1(6,1) > 1.2556*1e4*100)
    Xk1_k1(6,1) = single(1.2556*1e4*100);
elseif (Xk1_k1(6,1) < 1.2556*1e4/100)
    Xk1_k1(6,1) = single(1.2556*1e4/100);
end
X1_hat = Xk1_k1(1,1);X2_hat = Xk1_k1(2,1);
Theta1_hat = Xk1_k1(3,1);Theta2_hat = Xk1_k1(4,1);Theta3_hat = Xk1_k1(5,1);Theta4_hat = Xk1_k1(6,1);

== matlab function TEST_IPM_2_0/Subsystem1/MATLAB Function3 ==
  data: A input; Ldd output; B input; C input; Ldq output; Lqq output
function [Ldd,Ldq,Lqq] = inverse(A,B,C)
T = [C,B;B,A];
V = T^-1;
Ldd = V(1,1);
Ldq = V(1,2);
Lqq = V(2,2);
end

== matlab function TEST_IPM_2_0/INT/Extra Observer/MATLAB Function5 ==
  data: id input; iq input; ud input; uq input; kr input; kld input; klq input; flag_clear input; MRAS_Rs data_store_memory; MRAS_Ld data_store_memory; MRAS_Lq data_store_memory; MRAS_Idh data_store_memory; MRAS_Iqh data_store_memory
function MRAS(id,iq,ud,uq,kr,kld,klq,flag_clear)
global MRAS_Rs MRAS_Ld MRAS_Lq MRAS_Idh MRAS_Iqh
if(flag_clear == uint16(1))
    MRAS_Rs = single(14e3);
    MRAS_Ld = single(80);
    MRAS_Lq = single(280);
    MRAS_Idh = single(0);
    MRAS_Iqh = single(0);
end
Didh = (ud * single(1e6) - MRAS_Rs * MRAS_Idh)/MRAS_Ld;
Diqh = (uq * single(1e6) - MRAS_Rs * MRAS_Iqh)/MRAS_Lq;
Idh_New = MRAS_Idh + Didh * single(1e-4);
Iqh_New = MRAS_Iqh + Diqh * single(1e-4);

DRs = kr * ((id - MRAS_Idh) * MRAS_Idh + (iq - MRAS_Iqh) * MRAS_Iqh);
DLd = kld * ((id - MRAS_Idh) * (Idh_New - MRAS_Idh));
DLq = klq * ((iq - MRAS_Iqh) * (Iqh_New - MRAS_Iqh));

MRAS_Rs = MRAS_Rs + DRs * single(1e-4);
MRAS_Ld = MRAS_Ld + DLd * single(1e-4);
MRAS_Lq = MRAS_Lq + DLq * single(1e-4);
MRAS_Idh = MRAS_Idh + Didh * single(1e-4);
MRAS_Iqh = MRAS_Iqh + Diqh * single(1e-4);


if(MRAS_Rs < single(0))
    MRAS_Rs = single(0);
elseif(MRAS_Rs > single(50e3))
    MRAS_Rs = single(50e3);
end
if(MRAS_Ld < single(10))
    MRAS_Ld = single(10);
elseif(MRAS_Ld > single(200))
    MRAS_Ld = single(200);
end
if(MRAS_Lq < single(10))
    MRAS_Lq = single(10);
elseif(MRAS_Lq > single(500))
    MRAS_Lq = single(500);
end

end

== matlab function TEST_IPM_2_0/INT/Motor Control/TorqueMode/PID_n /MATLAB Function ==
  data: Limit input; Input input; Output output
function Output = Saturation(Limit,Input)
if(Input >= Limit)
    Output = Limit;
elseif(Input <= -Limit)
    Output = -Limit;
else
    Output = Input;
end

== matlab function TEST_IPM_2_0/UdcREF/Subsystem1/MATLAB Function ==
  data: Target input single; Output output; Step input single; LastOutput input single; STOP data_store_memory
function Output = RAMPCONTROL(Target,Step,LastOutput)
global STOP
if(LastOutput <= Target)
    Temp = LastOutput + Step;
else
    Temp = LastOutput - Step;
end
if (abs(Temp - Target) <= Step * 2)
    Temp = Target;
end
if(STOP ~= uint16(0))
    Temp = single(0);
end
    Output = Temp;
    
end

== matlab function TEST_IPM_2_0/INT/Motor Control/FbLMode/MATLAB Function ==
  data: x1 input; z1 output; x2 input; x3 input; speed input; Lq_norm input; Ld_norm input; Cdc_norm input; Rs_norm input; Phi_dm_norm input; v1_in input; v2_in input; FbL_Rs data_store_memory; FbL_Cdc data_store_memory; FbL_Ld data_store_memory; FbL_Lq data_store_memory; FbL_Phif data_store_memory; z2 output; z3 output; u1 output; u2 output; Rdc input; iq_muti input
function [z1,z2,z3,u1,u2] = fcn(x1, x2, x3, speed, Lq_norm, Ld_norm, Cdc_norm, Rs_norm, Phi_dm_norm, v1_in, v2_in,Rdc, iq_muti)
we = abs(speed)*2*pi/60*4+0.01;
z1 = 3/2*Lq_norm*x1*x1*iq_muti + 3/2*Ld_norm*x2*x2 + Cdc_norm*x3;
z2 = -3*Rs_norm*(x1*x1+x2*x2) - 3*we*(Ld_norm-Lq_norm)*x1*x2 - 3*we*Phi_dm_norm*x1 - 2/Rdc*x3;
%z3 = Ld_norm*x2;
z3 = x2;
%反馈调节
v1 = v1_in;
v2 = v2_in;
V = [v1;v2];
%输出变量代换
f1 = -Rs_norm/Lq_norm*x1 - we*Ld_norm/Lq_norm*x2 - we*Phi_dm_norm/Lq_norm;
f2 = -Rs_norm/Ld_norm*x2 + we*Lq_norm/Ld_norm*x1;
f3 = -2/Cdc_norm/Rdc*x3;
f = [f1 f2 f3];
g1 = [1/Lq_norm 0 -3/Cdc_norm*x1];
g2 = [0 1/Ld_norm -3/Cdc_norm*x2];
Jacob_LfS11 = [-6*Rs_norm*x1-3*we*(Ld_norm-Lq_norm)*x2-3*we*Phi_dm_norm;
    -6*Rs_norm*x2-3*we*(Ld_norm-Lq_norm)*x1;
    -2/Rdc
    ];
Jacob_S21 = [0;
    1;
    0
    ];
LfLfS11 = f*Jacob_LfS11;
Lg1LfS11 = g1*Jacob_LfS11;
Lg2LfS11 = g2*Jacob_LfS11;
LfS21 = f*Jacob_S21;
Lg1S21 = g1*Jacob_S21;
Lg2S21 = g2*Jacob_S21;
E = 1e-4*[Lg1LfS11 Lg2LfS11;Lg1S21 Lg2S21];
A = [LfLfS11;LfS21];
U = E^-1*(-1e-4*A+V);
u1 = U(1);
u2 = U(2);

== matlab function TEST_IPM_2_0/INT/Motor Control/FbLMode/MATLAB Function2 ==
  data: Phif6Amp input; y output; Phif6Pha input; speed input
function y = fcn(Phif6Amp, Phif6Pha, speed)
we = abs(speed)*2*pi/60*4+0.01;
persistent t
if isempty(t)
    t=single(0);
end
t = t + 6*we*1e-4;
if t >= 2*pi
    t = single(0);
end
y = Phif6Amp*sin(t+Phif6Pha/180*pi);

== matlab function TEST_IPM_2_0/INT/Motor Control/SVPWM/MATLAB Function1 ==
  data: theta_in input; theta_out output; controlmode input
function theta_out = fcn(theta_in, controlmode)
temp = theta_in;
if (temp > single(2*pi)) && (controlmode == uint16(3) || controlmode == uint16(6))
    temp = temp - single(2*pi);
end
theta_out = temp;

== matlab function TEST_IPM_2_0/INT/Motor Control/Current_PI/deadzone compesation/MATLAB Function3 ==
  data: I input; Uerror output; K input; Udead input
function Uerror = VSIComp(I,K,Udead)
% Uerror = single(2) * Udead * (single(1)/(single(1) + exp(-K*I))-single(0.5));
Uerror = Udead * atan( I * K ) /(single(pi) * single(0.5));
end

== matlab function TEST_IPM_2_0/INT/Motor Control/Current_PI/deadzone compesation/MATLAB Function5 ==
  data: I input; Uerror output; K input; Udead input
function Uerror = VSIComp(I,K,Udead)
% Uerror = single(2) * Udead * (single(1)/(single(1) + exp(-K*I))-single(0.5));
Uerror = Udead * atan( I * K ) /(single(pi) * single(0.5));
end

== matlab function TEST_IPM_2_0/INT/Motor Control/Current_PI/deadzone compesation/MATLAB Function6 ==
  data: I input; Uerror output; K input; Udead input
function Uerror = VSIComp(I,K,Udead)
% Uerror = single(2) * Udead * (single(1)/(single(1) + exp(-K*I))-single(0.5));
Uerror = Udead * atan( I * K ) /(single(pi) * single(0.5));
end
